simulink model "c00006M_harness"  (R2018a)
settings: Solver=ode3  StartTime=0.0  StopTime=10.0  RelTol=1e-3  EnableMultiTasking=on
undefined symbols (not defined in the file): b, DiscIntNeverNeededParam, J, K, L, PosMinimaW3, R, sigbuilder_block
(part 2 of 42)

== system c00006M_harness/CPSUT ==
  DW1 : Inport  OutMin=0  OutMax=4  OutDataTypeStr=int8
  DW2 : Inport  Port=2  OutMin=0  OutMax=4  OutDataTypeStr=int8
  DW3 : Inport  Port=3  OutMin=0  OutMax=4  OutDataTypeStr=int8
  P1W2 : Inport  Port=4  OutMin=0  OutMax=4  OutDataTypeStr=int8
  P2W3 : Inport  Port=5  OutMin=0  OutMax=4  OutDataTypeStr=int8
  O1 : Inport  Port=6  OutDataTypeStr=boolean
  O2 : Inport  Port=7  OutDataTypeStr=boolean
  O3 : Inport  Port=8  OutDataTypeStr=boolean
  CW3C : Inport  Port=9  OutMin=0  OutMax=4  OutDataTypeStr=int8
  Cyber : Subsystem
  M : Memory
  M1 : Memory
  M2 : Memory
  Physical : Subsystem
  S1 : Subsystem
  S2 : Subsystem
  S3 : Subsystem
  W1Pos : Outport
  W2Pos : Outport  Port=2
  W3Pos : Outport  Port=3
  wires:
  P2W3/1 -> Cyber/8(P2W3)
  S1/1(SensorOut) -> M/1
  CW3C/1 -> Cyber/12(CW3C)
  Physical/1(W1) -> W1Pos/1, S1/1(PhyMeasure)
  S3/1(SensorOut) -> M2/1
  O2/1 -> Cyber/10(OW2)
  Cyber/3(W3) -> Physical/3(InW3)
  O1/1 -> Cyber/9(OW1)
  Cyber/1(W1) -> Physical/1(InW1)
  Cyber/2(W2) -> Physical/2(InW2)
  M2/1 -> Cyber/3(PosW3)
  P1W2/1 -> Cyber/7(P1W2)
  O3/1 -> Cyber/11(OW3)
  DW3/1 -> Cyber/6(DW3)
  M1/1 -> Cyber/2(PosW2)
  Physical/3(W3) -> W3Pos/1, S3/1(PhyMeasure)
  M/1 -> Cyber/1(PosW1)
  DW1/1 -> Cyber/4(DW1)
  Physical/2(W2) -> W2Pos/1, S2/1(PhyMeasure)
  S2/1(SensorOut) -> M1/1
  DW2/1 -> Cyber/5(DW2)

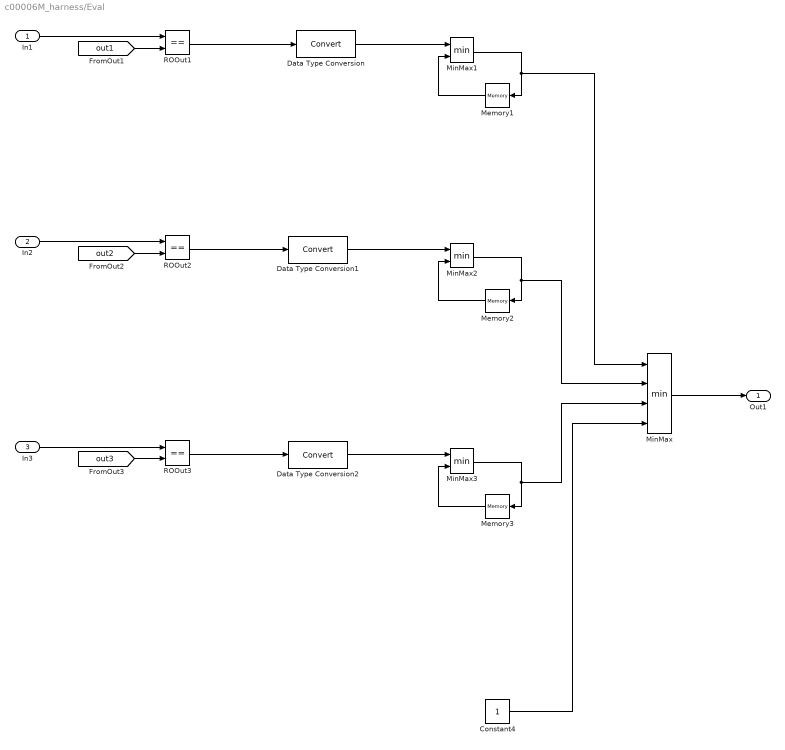
== system c00006M_harness/Eval ==
  In1 : Inport
  In2 : Inport  Port=2
  In3 : Inport  Port=3
  Constant4 : Constant
  Data Type Conversion : DataTypeConversion
  Data Type Conversion1 : DataTypeConversion
  Data Type Conversion2 : DataTypeConversion
  Memory1 : Memory  InitialCondition=1
  Memory2 : Memory  InitialCondition=1
  Memory3 : Memory  InitialCondition=1
  MinMax : MinMax  Inputs=4
  MinMax1 : MinMax  Inputs=2
  MinMax2 : MinMax  Inputs=2
  MinMax3 : MinMax  Inputs=2
  ROOut1 : RelationalOperator  Operator===  OutDataTypeStr=boolean  RndMeth=Simplest
  ROOut2 : RelationalOperator  Operator===  OutDataTypeStr=boolean  RndMeth=Simplest
  ROOut3 : RelationalOperator  Operator===  OutDataTypeStr=boolean  RndMeth=Simplest
  Out1 : Outport
  wires:
  MinMax/1 -> Out1/1
  [out3] -> ROOut3/2
  In3/1 -> ROOut3/1
  [out1] -> ROOut1/2
  In2/1 -> ROOut2/1
  In1/1 -> ROOut1/1
  [out2] -> ROOut2/2
  Memory1/1 -> MinMax1/2
  MinMax3/1 -> MinMax/3, Memory3/1
  ROOut3/1 -> Data Type Conversion2/1
  ROOut2/1 -> Data Type Conversion1/1
  Memory3/1 -> MinMax3/2
  Memory2/1 -> MinMax2/2
  ROOut1/1 -> Data Type Conversion/1
  MinMax2/1 -> MinMax/2, Memory2/1
  MinMax1/1 -> MinMax/1, Memory1/1
  Data Type Conversion/1 -> MinMax1/1
  Data Type Conversion1/1 -> MinMax2/1
  Data Type Conversion2/1 -> MinMax3/1
  Constant4/1 -> MinMax/4

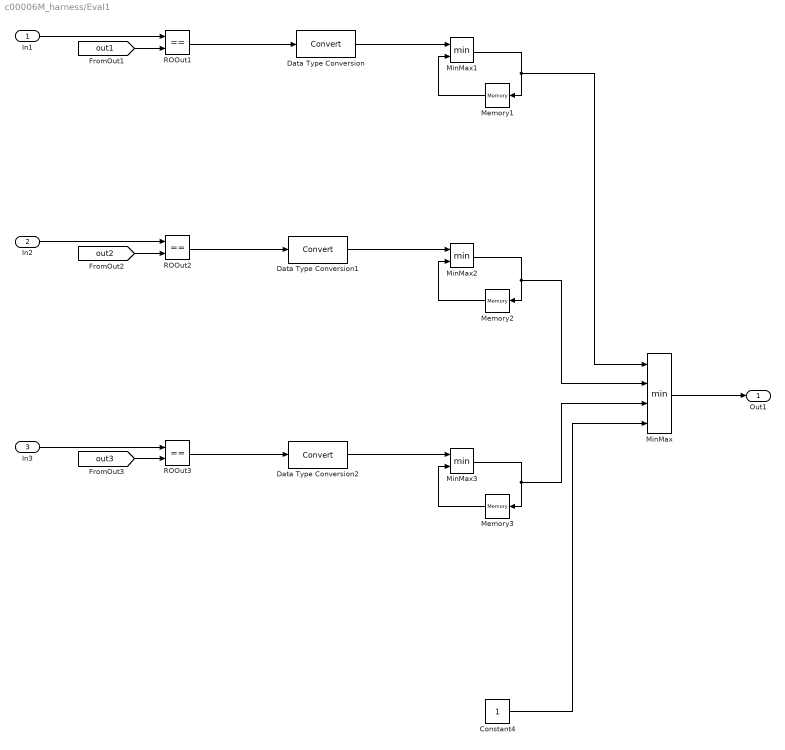
== system c00006M_harness/Eval1 ==
  In1 : Inport
  In2 : Inport  Port=2
  In3 : Inport  Port=3
  Constant4 : Constant
  Data Type Conversion : DataTypeConversion
  Data Type Conversion1 : DataTypeConversion
  Data Type Conversion2 : DataTypeConversion
  Memory1 : Memory  InitialCondition=1
  Memory2 : Memory  InitialCondition=1
  Memory3 : Memory  InitialCondition=1
  MinMax : MinMax  Inputs=4
  MinMax1 : MinMax  Inputs=2
  MinMax2 : MinMax  Inputs=2
  MinMax3 : MinMax  Inputs=2
  ROOut1 : RelationalOperator  Operator===  OutDataTypeStr=boolean  RndMeth=Simplest
  ROOut2 : RelationalOperator  Operator===  OutDataTypeStr=boolean  RndMeth=Simplest
  ROOut3 : RelationalOperator  Operator===  OutDataTypeStr=boolean  RndMeth=Simplest
  Out1 : Outport
  wires:
  Data Type Conversion2/1 -> MinMax3/1
  Data Type Conversion1/1 -> MinMax2/1
  Data Type Conversion/1 -> MinMax1/1
  MinMax1/1 -> Memory1/1, MinMax/1
  MinMax2/1 -> Memory2/1, MinMax/2
  ROOut1/1 -> Data Type Conversion/1
  Memory2/1 -> MinMax2/2
  Memory3/1 -> MinMax3/2
  ROOut2/1 -> Data Type Conversion1/1
  ROOut3/1 -> Data Type Conversion2/1
  MinMax3/1 -> Memory3/1, MinMax/3
  Memory1/1 -> MinMax1/2
  [out2] -> ROOut2/2
  In1/1 -> ROOut1/1
  In2/1 -> ROOut2/1
  [out1] -> ROOut1/2
  In3/1 -> ROOut3/1
  [out3] -> ROOut3/2
  MinMax/1 -> Out1/1
  Constant4/1 -> MinMax/4

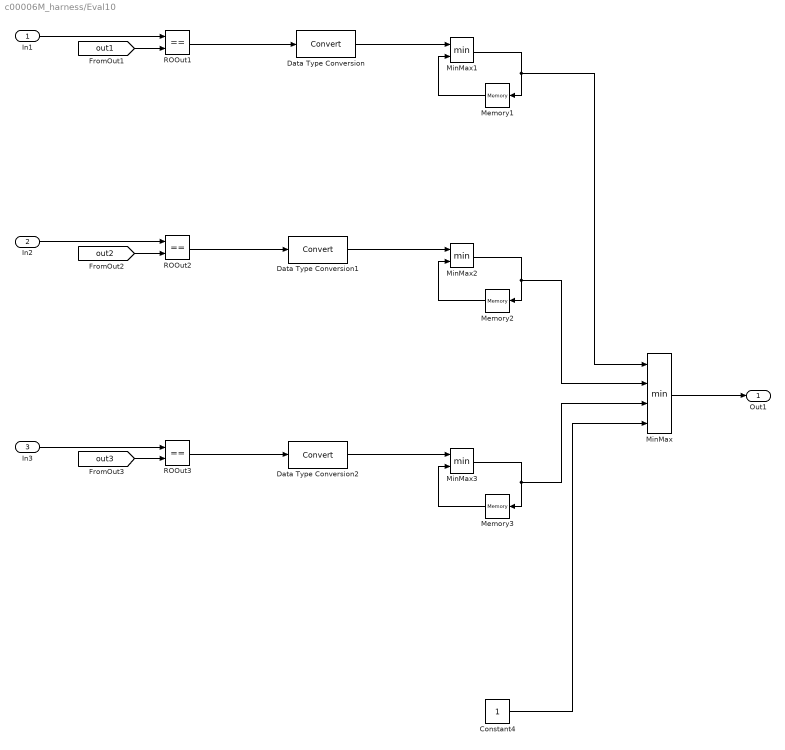
== system c00006M_harness/Eval10 ==
  In1 : Inport
  In2 : Inport  Port=2
  In3 : Inport  Port=3
  Constant4 : Constant
  Data Type Conversion : DataTypeConversion
  Data Type Conversion1 : DataTypeConversion
  Data Type Conversion2 : DataTypeConversion
  Memory1 : Memory  InitialCondition=1
  Memory2 : Memory  InitialCondition=1
  Memory3 : Memory  InitialCondition=1
  MinMax : MinMax  Inputs=4
  MinMax1 : MinMax  Inputs=2
  MinMax2 : MinMax  Inputs=2
  MinMax3 : MinMax  Inputs=2
  ROOut1 : RelationalOperator  Operator===  OutDataTypeStr=boolean  RndMeth=Simplest
  ROOut2 : RelationalOperator  Operator===  OutDataTypeStr=boolean  RndMeth=Simplest
  ROOut3 : RelationalOperator  Operator===  OutDataTypeStr=boolean  RndMeth=Simplest
  Out1 : Outport
  wires:
  Data Type Conversion2/1 -> MinMax3/1
  Data Type Conversion1/1 -> MinMax2/1
  Data Type Conversion/1 -> MinMax1/1
  MinMax1/1 -> Memory1/1, MinMax/1
  MinMax2/1 -> Memory2/1, MinMax/2
  ROOut1/1 -> Data Type Conversion/1
  Memory2/1 -> MinMax2/2
  Memory3/1 -> MinMax3/2
  ROOut2/1 -> Data Type Conversion1/1
  ROOut3/1 -> Data Type Conversion2/1
  MinMax3/1 -> Memory3/1, MinMax/3
  Memory1/1 -> MinMax1/2
  [out2] -> ROOut2/2
  In1/1 -> ROOut1/1
  In2/1 -> ROOut2/1
  [out1] -> ROOut1/2
  In3/1 -> ROOut3/1
  [out3] -> ROOut3/2
  MinMax/1 -> Out1/1
  Constant4/1 -> MinMax/4

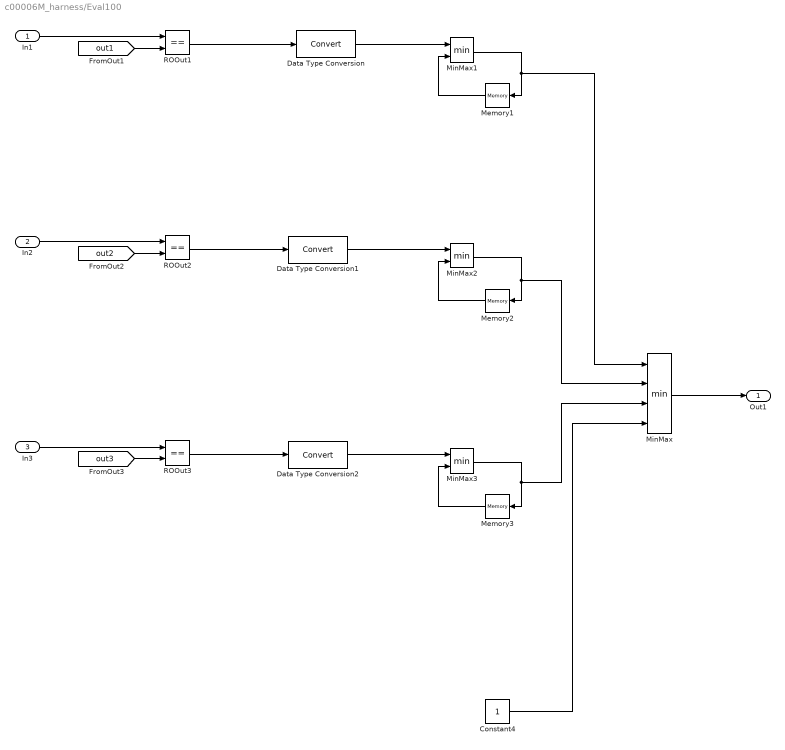
== system c00006M_harness/Eval100 ==
  In1 : Inport
  In2 : Inport  Port=2
  In3 : Inport  Port=3
  Constant4 : Constant
  Data Type Conversion : DataTypeConversion
  Data Type Conversion1 : DataTypeConversion
  Data Type Conversion2 : DataTypeConversion
  Memory1 : Memory  InitialCondition=1
  Memory2 : Memory  InitialCondition=1
  Memory3 : Memory  InitialCondition=1
  MinMax : MinMax  Inputs=4
  MinMax1 : MinMax  Inputs=2
  MinMax2 : MinMax  Inputs=2
  MinMax3 : MinMax  Inputs=2
  ROOut1 : RelationalOperator  Operator===  OutDataTypeStr=boolean  RndMeth=Simplest
  ROOut2 : RelationalOperator  Operator===  OutDataTypeStr=boolean  RndMeth=Simplest
  ROOut3 : RelationalOperator  Operator===  OutDataTypeStr=boolean  RndMeth=Simplest
  Out1 : Outport
  wires:
  Data Type Conversion2/1 -> MinMax3/1
  Data Type Conversion1/1 -> MinMax2/1
  Data Type Conversion/1 -> MinMax1/1
  MinMax1/1 -> Memory1/1, MinMax/1
  MinMax2/1 -> Memory2/1, MinMax/2
  ROOut1/1 -> Data Type Conversion/1
  Memory2/1 -> MinMax2/2
  Memory3/1 -> MinMax3/2
  ROOut2/1 -> Data Type Conversion1/1
  ROOut3/1 -> Data Type Conversion2/1
  MinMax3/1 -> Memory3/1, MinMax/3
  Memory1/1 -> MinMax1/2
  [out2] -> ROOut2/2
  In1/1 -> ROOut1/1
  In2/1 -> ROOut2/1
  [out1] -> ROOut1/2
  In3/1 -> ROOut3/1
  [out3] -> ROOut3/2
  MinMax/1 -> Out1/1
  Constant4/1 -> MinMax/4

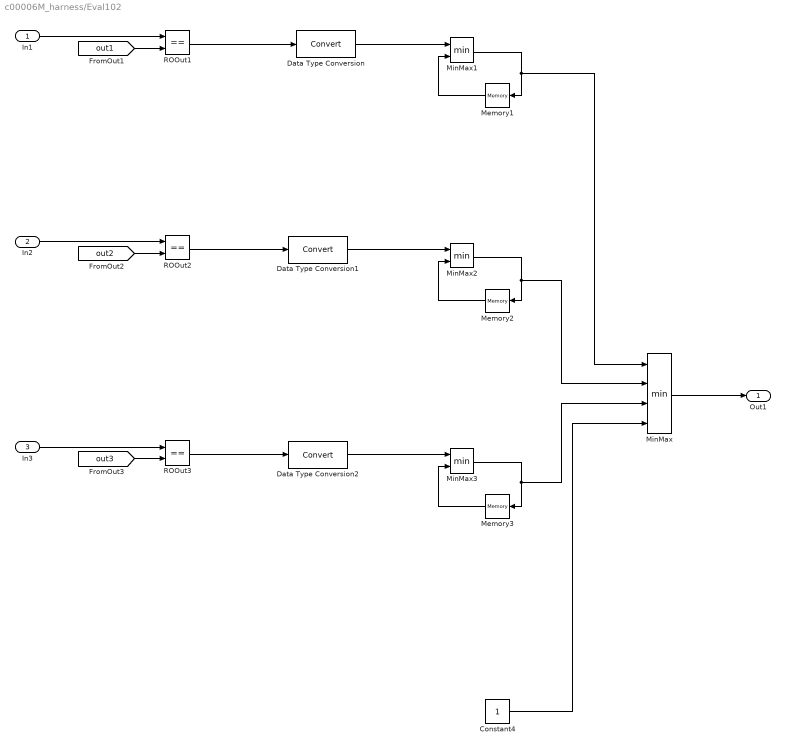
== system c00006M_harness/Eval102 ==
  In1 : Inport
  In2 : Inport  Port=2
  In3 : Inport  Port=3
  Constant4 : Constant
  Data Type Conversion : DataTypeConversion
  Data Type Conversion1 : DataTypeConversion
  Data Type Conversion2 : DataTypeConversion
  Memory1 : Memory  InitialCondition=1
  Memory2 : Memory  InitialCondition=1
  Memory3 : Memory  InitialCondition=1
  MinMax : MinMax  Inputs=4
  MinMax1 : MinMax  Inputs=2
  MinMax2 : MinMax  Inputs=2
  MinMax3 : MinMax  Inputs=2
  ROOut1 : RelationalOperator  Operator===  OutDataTypeStr=boolean  RndMeth=Simplest
  ROOut2 : RelationalOperator  Operator===  OutDataTypeStr=boolean  RndMeth=Simplest
  ROOut3 : RelationalOperator  Operator===  OutDataTypeStr=boolean  RndMeth=Simplest
  Out1 : Outport
  wires:
  Data Type Conversion2/1 -> MinMax3/1
  Data Type Conversion1/1 -> MinMax2/1
  Data Type Conversion/1 -> MinMax1/1
  MinMax1/1 -> Memory1/1, MinMax/1
  MinMax2/1 -> Memory2/1, MinMax/2
  ROOut1/1 -> Data Type Conversion/1
  Memory2/1 -> MinMax2/2
  Memory3/1 -> MinMax3/2
  ROOut2/1 -> Data Type Conversion1/1
  ROOut3/1 -> Data Type Conversion2/1
  MinMax3/1 -> Memory3/1, MinMax/3
  Memory1/1 -> MinMax1/2
  [out2] -> ROOut2/2
  In1/1 -> ROOut1/1
  In2/1 -> ROOut2/1
  [out1] -> ROOut1/2
  In3/1 -> ROOut3/1
  [out3] -> ROOut3/2
  MinMax/1 -> Out1/1
  Constant4/1 -> MinMax/4

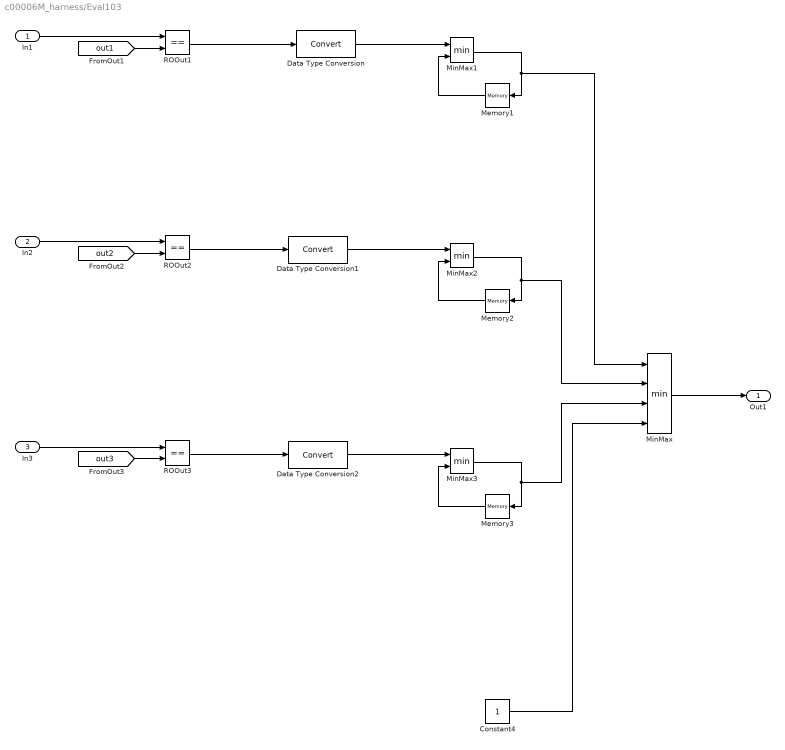
== system c00006M_harness/Eval103 ==
  In1 : Inport
  In2 : Inport  Port=2
  In3 : Inport  Port=3
  Constant4 : Constant
  Data Type Conversion : DataTypeConversion
  Data Type Conversion1 : DataTypeConversion
  Data Type Conversion2 : DataTypeConversion
  Memory1 : Memory  InitialCondition=1
  Memory2 : Memory  InitialCondition=1
  Memory3 : Memory  InitialCondition=1
  MinMax : MinMax  Inputs=4
  MinMax1 : MinMax  Inputs=2
  MinMax2 : MinMax  Inputs=2
  MinMax3 : MinMax  Inputs=2
  ROOut1 : RelationalOperator  Operator===  OutDataTypeStr=boolean  RndMeth=Simplest
  ROOut2 : RelationalOperator  Operator===  OutDataTypeStr=boolean  RndMeth=Simplest
  ROOut3 : RelationalOperator  Operator===  OutDataTypeStr=boolean  RndMeth=Simplest
  Out1 : Outport
  wires:
  Data Type Conversion2/1 -> MinMax3/1
  Data Type Conversion1/1 -> MinMax2/1
  Data Type Conversion/1 -> MinMax1/1
  MinMax1/1 -> Memory1/1, MinMax/1
  MinMax2/1 -> Memory2/1, MinMax/2
  ROOut1/1 -> Data Type Conversion/1
  Memory2/1 -> MinMax2/2
  Memory3/1 -> MinMax3/2
  ROOut2/1 -> Data Type Conversion1/1
  ROOut3/1 -> Data Type Conversion2/1
  MinMax3/1 -> Memory3/1, MinMax/3
  Memory1/1 -> MinMax1/2
  [out2] -> ROOut2/2
  In1/1 -> ROOut1/1
  In2/1 -> ROOut2/1
  [out1] -> ROOut1/2
  In3/1 -> ROOut3/1
  [out3] -> ROOut3/2
  MinMax/1 -> Out1/1
  Constant4/1 -> MinMax/4

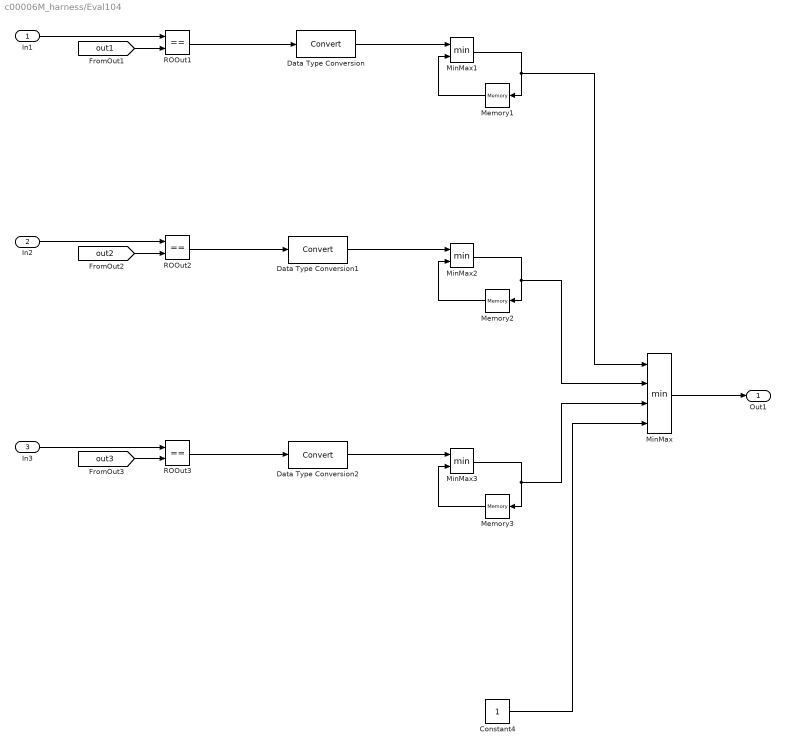
== system c00006M_harness/Eval104 ==
  In1 : Inport
  In2 : Inport  Port=2
  In3 : Inport  Port=3
  Constant4 : Constant
  Data Type Conversion : DataTypeConversion
  Data Type Conversion1 : DataTypeConversion
  Data Type Conversion2 : DataTypeConversion
  Memory1 : Memory  InitialCondition=1
  Memory2 : Memory  InitialCondition=1
  Memory3 : Memory  InitialCondition=1
  MinMax : MinMax  Inputs=4
  MinMax1 : MinMax  Inputs=2
  MinMax2 : MinMax  Inputs=2
  MinMax3 : MinMax  Inputs=2
  ROOut1 : RelationalOperator  Operator===  OutDataTypeStr=boolean  RndMeth=Simplest
  ROOut2 : RelationalOperator  Operator===  OutDataTypeStr=boolean  RndMeth=Simplest
  ROOut3 : RelationalOperator  Operator===  OutDataTypeStr=boolean  RndMeth=Simplest
  Out1 : Outport
  wires:
  Data Type Conversion2/1 -> MinMax3/1
  Data Type Conversion1/1 -> MinMax2/1
  Data Type Conversion/1 -> MinMax1/1
  MinMax1/1 -> Memory1/1, MinMax/1
  MinMax2/1 -> Memory2/1, MinMax/2
  ROOut1/1 -> Data Type Conversion/1
  Memory2/1 -> MinMax2/2
  Memory3/1 -> MinMax3/2
  ROOut2/1 -> Data Type Conversion1/1
  ROOut3/1 -> Data Type Conversion2/1
  MinMax3/1 -> Memory3/1, MinMax/3
  Memory1/1 -> MinMax1/2
  [out2] -> ROOut2/2
  In1/1 -> ROOut1/1
  In2/1 -> ROOut2/1
  [out1] -> ROOut1/2
  In3/1 -> ROOut3/1
  [out3] -> ROOut3/2
  MinMax/1 -> Out1/1
  Constant4/1 -> MinMax/4

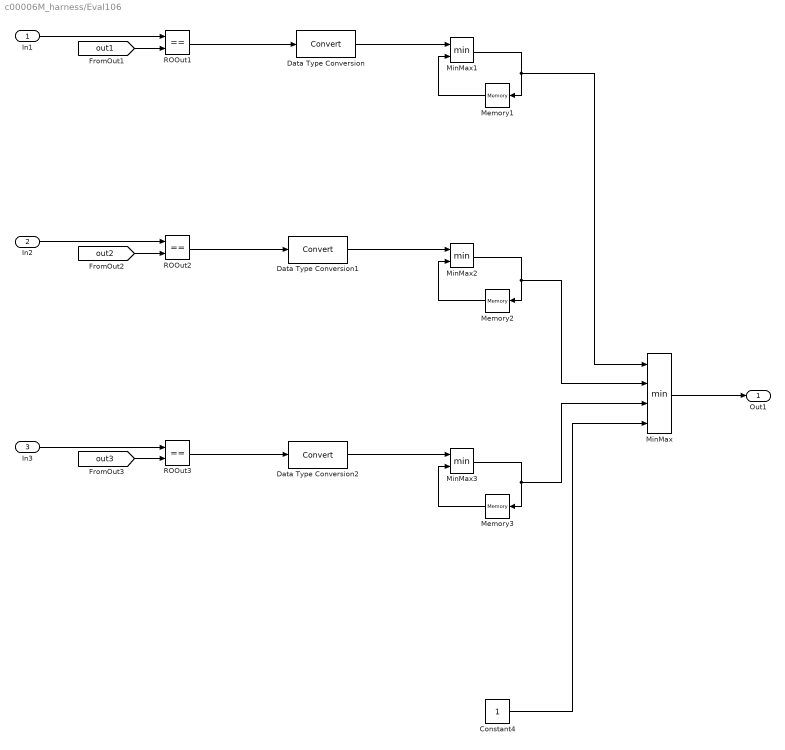
== system c00006M_harness/Eval106 ==
  In1 : Inport
  In2 : Inport  Port=2
  In3 : Inport  Port=3
  Constant4 : Constant
  Data Type Conversion : DataTypeConversion
  Data Type Conversion1 : DataTypeConversion
  Data Type Conversion2 : DataTypeConversion
  Memory1 : Memory  InitialCondition=1
  Memory2 : Memory  InitialCondition=1
  Memory3 : Memory  InitialCondition=1
  MinMax : MinMax  Inputs=4
  MinMax1 : MinMax  Inputs=2
  MinMax2 : MinMax  Inputs=2
  MinMax3 : MinMax  Inputs=2
  ROOut1 : RelationalOperator  Operator===  OutDataTypeStr=boolean  RndMeth=Simplest
  ROOut2 : RelationalOperator  Operator===  OutDataTypeStr=boolean  RndMeth=Simplest
  ROOut3 : RelationalOperator  Operator===  OutDataTypeStr=boolean  RndMeth=Simplest
  Out1 : Outport
  wires:
  Data Type Conversion2/1 -> MinMax3/1
  Data Type Conversion1/1 -> MinMax2/1
  Data Type Conversion/1 -> MinMax1/1
  MinMax1/1 -> Memory1/1, MinMax/1
  MinMax2/1 -> Memory2/1, MinMax/2
  ROOut1/1 -> Data Type Conversion/1
  Memory2/1 -> MinMax2/2
  Memory3/1 -> MinMax3/2
  ROOut2/1 -> Data Type Conversion1/1
  ROOut3/1 -> Data Type Conversion2/1
  MinMax3/1 -> Memory3/1, MinMax/3
  Memory1/1 -> MinMax1/2
  [out2] -> ROOut2/2
  In1/1 -> ROOut1/1
  In2/1 -> ROOut2/1
  [out1] -> ROOut1/2
  In3/1 -> ROOut3/1
  [out3] -> ROOut3/2
  MinMax/1 -> Out1/1
  Constant4/1 -> MinMax/4

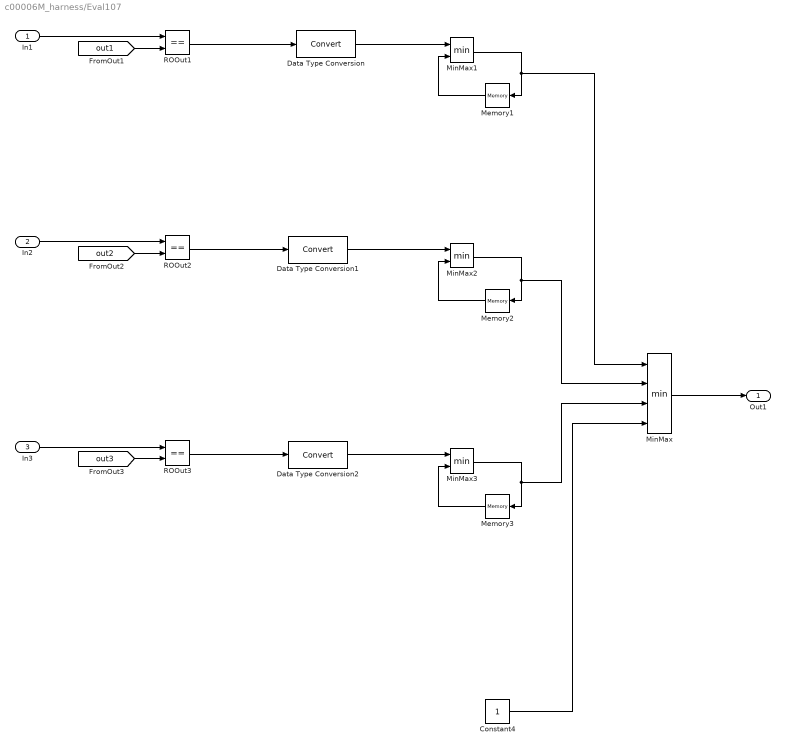
== system c00006M_harness/Eval107 ==
  In1 : Inport
  In2 : Inport  Port=2
  In3 : Inport  Port=3
  Constant4 : Constant
  Data Type Conversion : DataTypeConversion
  Data Type Conversion1 : DataTypeConversion
  Data Type Conversion2 : DataTypeConversion
  Memory1 : Memory  InitialCondition=1
  Memory2 : Memory  InitialCondition=1
  Memory3 : Memory  InitialCondition=1
  MinMax : MinMax  Inputs=4
  MinMax1 : MinMax  Inputs=2
  MinMax2 : MinMax  Inputs=2
  MinMax3 : MinMax  Inputs=2
  ROOut1 : RelationalOperator  Operator===  OutDataTypeStr=boolean  RndMeth=Simplest
  ROOut2 : RelationalOperator  Operator===  OutDataTypeStr=boolean  RndMeth=Simplest
  ROOut3 : RelationalOperator  Operator===  OutDataTypeStr=boolean  RndMeth=Simplest
  Out1 : Outport
  wires:
  Data Type Conversion2/1 -> MinMax3/1
  Data Type Conversion1/1 -> MinMax2/1
  Data Type Conversion/1 -> MinMax1/1
  MinMax1/1 -> Memory1/1, MinMax/1
  MinMax2/1 -> Memory2/1, MinMax/2
  ROOut1/1 -> Data Type Conversion/1
  Memory2/1 -> MinMax2/2
  Memory3/1 -> MinMax3/2
  ROOut2/1 -> Data Type Conversion1/1
  ROOut3/1 -> Data Type Conversion2/1
  MinMax3/1 -> Memory3/1, MinMax/3
  Memory1/1 -> MinMax1/2
  [out2] -> ROOut2/2
  In1/1 -> ROOut1/1
  In2/1 -> ROOut2/1
  [out1] -> ROOut1/2
  In3/1 -> ROOut3/1
  [out3] -> ROOut3/2
  MinMax/1 -> Out1/1
  Constant4/1 -> MinMax/4

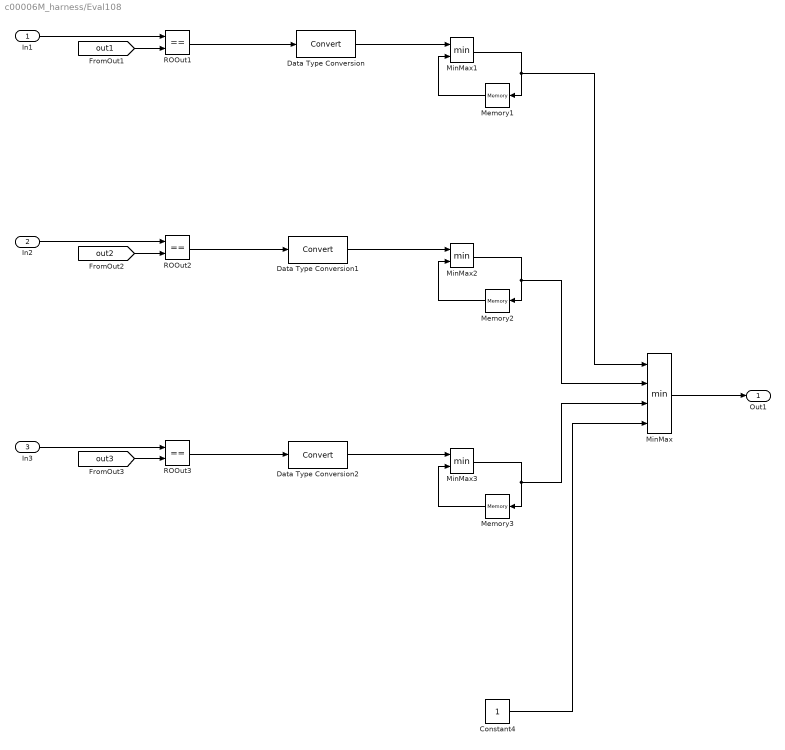
== system c00006M_harness/Eval108 ==
  In1 : Inport
  In2 : Inport  Port=2
  In3 : Inport  Port=3
  Constant4 : Constant
  Data Type Conversion : DataTypeConversion
  Data Type Conversion1 : DataTypeConversion
  Data Type Conversion2 : DataTypeConversion
  Memory1 : Memory  InitialCondition=1
  Memory2 : Memory  InitialCondition=1
  Memory3 : Memory  InitialCondition=1
  MinMax : MinMax  Inputs=4
  MinMax1 : MinMax  Inputs=2
  MinMax2 : MinMax  Inputs=2
  MinMax3 : MinMax  Inputs=2
  ROOut1 : RelationalOperator  Operator===  OutDataTypeStr=boolean  RndMeth=Simplest
  ROOut2 : RelationalOperator  Operator===  OutDataTypeStr=boolean  RndMeth=Simplest
  ROOut3 : RelationalOperator  Operator===  OutDataTypeStr=boolean  RndMeth=Simplest
  Out1 : Outport
  wires:
  Data Type Conversion2/1 -> MinMax3/1
  Data Type Conversion1/1 -> MinMax2/1
  Data Type Conversion/1 -> MinMax1/1
  MinMax1/1 -> Memory1/1, MinMax/1
  MinMax2/1 -> Memory2/1, MinMax/2
  ROOut1/1 -> Data Type Conversion/1
  Memory2/1 -> MinMax2/2
  Memory3/1 -> MinMax3/2
  ROOut2/1 -> Data Type Conversion1/1
  ROOut3/1 -> Data Type Conversion2/1
  MinMax3/1 -> Memory3/1, MinMax/3
  Memory1/1 -> MinMax1/2
  [out2] -> ROOut2/2
  In1/1 -> ROOut1/1
  In2/1 -> ROOut2/1
  [out1] -> ROOut1/2
  In3/1 -> ROOut3/1
  [out3] -> ROOut3/2
  MinMax/1 -> Out1/1
  Constant4/1 -> MinMax/4

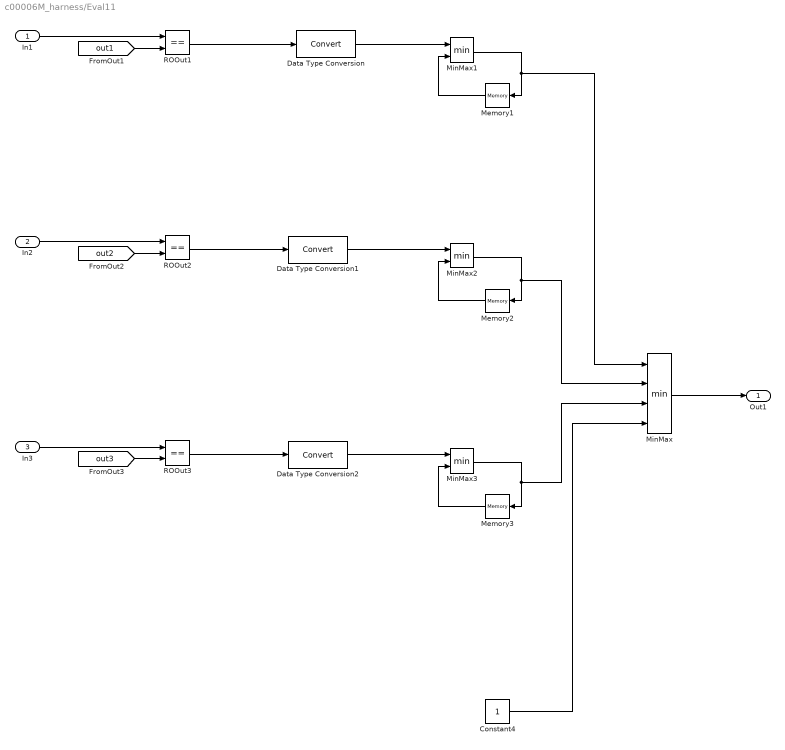
== system c00006M_harness/Eval11 ==
  In1 : Inport
  In2 : Inport  Port=2
  In3 : Inport  Port=3
  Constant4 : Constant
  Data Type Conversion : DataTypeConversion
  Data Type Conversion1 : DataTypeConversion
  Data Type Conversion2 : DataTypeConversion
  Memory1 : Memory  InitialCondition=1
  Memory2 : Memory  InitialCondition=1
  Memory3 : Memory  InitialCondition=1
  MinMax : MinMax  Inputs=4
  MinMax1 : MinMax  Inputs=2
  MinMax2 : MinMax  Inputs=2
  MinMax3 : MinMax  Inputs=2
  ROOut1 : RelationalOperator  Operator===  OutDataTypeStr=boolean  RndMeth=Simplest
  ROOut2 : RelationalOperator  Operator===  OutDataTypeStr=boolean  RndMeth=Simplest
  ROOut3 : RelationalOperator  Operator===  OutDataTypeStr=boolean  RndMeth=Simplest
  Out1 : Outport
  wires:
  Data Type Conversion2/1 -> MinMax3/1
  Data Type Conversion1/1 -> MinMax2/1
  Data Type Conversion/1 -> MinMax1/1
  MinMax1/1 -> Memory1/1, MinMax/1
  MinMax2/1 -> Memory2/1, MinMax/2
  ROOut1/1 -> Data Type Conversion/1
  Memory2/1 -> MinMax2/2
  Memory3/1 -> MinMax3/2
  ROOut2/1 -> Data Type Conversion1/1
  ROOut3/1 -> Data Type Conversion2/1
  MinMax3/1 -> Memory3/1, MinMax/3
  Memory1/1 -> MinMax1/2
  [out2] -> ROOut2/2
  In1/1 -> ROOut1/1
  In2/1 -> ROOut2/1
  [out1] -> ROOut1/2
  In3/1 -> ROOut3/1
  [out3] -> ROOut3/2
  MinMax/1 -> Out1/1
  Constant4/1 -> MinMax/4

== system c00006M_harness/Eval110 ==
  In1 : Inport
  In2 : Inport  Port=2
  In3 : Inport  Port=3
  Constant4 : Constant
  Data Type Conversion : DataTypeConversion
  Data Type Conversion1 : DataTypeConversion
  Data Type Conversion2 : DataTypeConversion
  Memory1 : Memory  InitialCondition=1
  Memory2 : Memory  InitialCondition=1
  Memory3 : Memory  InitialCondition=1
  MinMax : MinMax  Inputs=4
  MinMax1 : MinMax  Inputs=2
  MinMax2 : MinMax  Inputs=2
  MinMax3 : MinMax  Inputs=2
  ROOut1 : RelationalOperator  Operator===  OutDataTypeStr=boolean  RndMeth=Simplest
  ROOut2 : RelationalOperator  Operator===  OutDataTypeStr=boolean  RndMeth=Simplest
  ROOut3 : RelationalOperator  Operator===  OutDataTypeStr=boolean  RndMeth=Simplest
  Out1 : Outport
  wires:
  Data Type Conversion2/1 -> MinMax3/1
  Data Type Conversion1/1 -> MinMax2/1
  Data Type Conversion/1 -> MinMax1/1
  MinMax1/1 -> Memory1/1, MinMax/1
  MinMax2/1 -> Memory2/1, MinMax/2
  ROOut1/1 -> Data Type Conversion/1
  Memory2/1 -> MinMax2/2
  Memory3/1 -> MinMax3/2
  ROOut2/1 -> Data Type Conversion1/1
  ROOut3/1 -> Data Type Conversion2/1
  MinMax3/1 -> Memory3/1, MinMax/3
  Memory1/1 -> MinMax1/2
  [out2] -> ROOut2/2
  In1/1 -> ROOut1/1
  In2/1 -> ROOut2/1
  [out1] -> ROOut1/2
  In3/1 -> ROOut3/1
  [out3] -> ROOut3/2
  MinMax/1 -> Out1/1
  Constant4/1 -> MinMax/4

== system c00006M_harness/Eval111 ==
  In1 : Inport
  In2 : Inport  Port=2
  In3 : Inport  Port=3
  Constant4 : Constant
  Data Type Conversion : DataTypeConversion
  Data Type Conversion1 : DataTypeConversion
  Data Type Conversion2 : DataTypeConversion
  Memory1 : Memory  InitialCondition=1
  Memory2 : Memory  InitialCondition=1
  Memory3 : Memory  InitialCondition=1
  MinMax : MinMax  Inputs=4
  MinMax1 : MinMax  Inputs=2
  MinMax2 : MinMax  Inputs=2
  MinMax3 : MinMax  Inputs=2
  ROOut1 : RelationalOperator  Operator===  OutDataTypeStr=boolean  RndMeth=Simplest
  ROOut2 : RelationalOperator  Operator===  OutDataTypeStr=boolean  RndMeth=Simplest
  ROOut3 : RelationalOperator  Operator===  OutDataTypeStr=boolean  RndMeth=Simplest
  Out1 : Outport
  wires:
  Data Type Conversion2/1 -> MinMax3/1
  Data Type Conversion1/1 -> MinMax2/1
  Data Type Conversion/1 -> MinMax1/1
  MinMax1/1 -> Memory1/1, MinMax/1
  MinMax2/1 -> Memory2/1, MinMax/2
  ROOut1/1 -> Data Type Conversion/1
  Memory2/1 -> MinMax2/2
  Memory3/1 -> MinMax3/2
  ROOut2/1 -> Data Type Conversion1/1
  ROOut3/1 -> Data Type Conversion2/1
  MinMax3/1 -> Memory3/1, MinMax/3
  Memory1/1 -> MinMax1/2
  [out2] -> ROOut2/2
  In1/1 -> ROOut1/1
  In2/1 -> ROOut2/1
  [out1] -> ROOut1/2
  In3/1 -> ROOut3/1
  [out3] -> ROOut3/2
  MinMax/1 -> Out1/1
  Constant4/1 -> MinMax/4

== system c00006M_harness/Eval112 ==
  In1 : Inport
  In2 : Inport  Port=2
  In3 : Inport  Port=3
  Constant4 : Constant
  Data Type Conversion : DataTypeConversion
  Data Type Conversion1 : DataTypeConversion
  Data Type Conversion2 : DataTypeConversion
  Memory1 : Memory  InitialCondition=1
  Memory2 : Memory  InitialCondition=1
  Memory3 : Memory  InitialCondition=1
  MinMax : MinMax  Inputs=4
  MinMax1 : MinMax  Inputs=2
  MinMax2 : MinMax  Inputs=2
  MinMax3 : MinMax  Inputs=2
  ROOut1 : RelationalOperator  Operator===  OutDataTypeStr=boolean  RndMeth=Simplest
  ROOut2 : RelationalOperator  Operator===  OutDataTypeStr=boolean  RndMeth=Simplest
  ROOut3 : RelationalOperator  Operator===  OutDataTypeStr=boolean  RndMeth=Simplest
  Out1 : Outport
  wires:
  Data Type Conversion2/1 -> MinMax3/1
  Data Type Conversion1/1 -> MinMax2/1
  Data Type Conversion/1 -> MinMax1/1
  MinMax1/1 -> Memory1/1, MinMax/1
  MinMax2/1 -> Memory2/1, MinMax/2
  ROOut1/1 -> Data Type Conversion/1
  Memory2/1 -> MinMax2/2
  Memory3/1 -> MinMax3/2
  ROOut2/1 -> Data Type Conversion1/1
  ROOut3/1 -> Data Type Conversion2/1
  MinMax3/1 -> Memory3/1, MinMax/3
  Memory1/1 -> MinMax1/2
  [out2] -> ROOut2/2
  In1/1 -> ROOut1/1
  In2/1 -> ROOut2/1
  [out1] -> ROOut1/2
  In3/1 -> ROOut3/1
  [out3] -> ROOut3/2
  MinMax/1 -> Out1/1
  Constant4/1 -> MinMax/4

== system c00006M_harness/Eval114 ==
  In1 : Inport
  In2 : Inport  Port=2
  In3 : Inport  Port=3
  Constant4 : Constant
  Data Type Conversion : DataTypeConversion
  Data Type Conversion1 : DataTypeConversion
  Data Type Conversion2 : DataTypeConversion
  Memory1 : Memory  InitialCondition=1
  Memory2 : Memory  InitialCondition=1
  Memory3 : Memory  InitialCondition=1
  MinMax : MinMax  Inputs=4
  MinMax1 : MinMax  Inputs=2
  MinMax2 : MinMax  Inputs=2
  MinMax3 : MinMax  Inputs=2
  ROOut1 : RelationalOperator  Operator===  OutDataTypeStr=boolean  RndMeth=Simplest
  ROOut2 : RelationalOperator  Operator===  OutDataTypeStr=boolean  RndMeth=Simplest
  ROOut3 : RelationalOperator  Operator===  OutDataTypeStr=boolean  RndMeth=Simplest
  Out1 : Outport
  wires:
  Data Type Conversion2/1 -> MinMax3/1
  Data Type Conversion1/1 -> MinMax2/1
  Data Type Conversion/1 -> MinMax1/1
  MinMax1/1 -> Memory1/1, MinMax/1
  MinMax2/1 -> Memory2/1, MinMax/2
  ROOut1/1 -> Data Type Conversion/1
  Memory2/1 -> MinMax2/2
  Memory3/1 -> MinMax3/2
  ROOut2/1 -> Data Type Conversion1/1
  ROOut3/1 -> Data Type Conversion2/1
  MinMax3/1 -> Memory3/1, MinMax/3
  Memory1/1 -> MinMax1/2
  [out2] -> ROOut2/2
  In1/1 -> ROOut1/1
  In2/1 -> ROOut2/1
  [out1] -> ROOut1/2
  In3/1 -> ROOut3/1
  [out3] -> ROOut3/2
  MinMax/1 -> Out1/1
  Constant4/1 -> MinMax/4

== system c00006M_harness/Eval115 ==
  In1 : Inport
  In2 : Inport  Port=2
  In3 : Inport  Port=3
  Constant4 : Constant
  Data Type Conversion : DataTypeConversion
  Data Type Conversion1 : DataTypeConversion
  Data Type Conversion2 : DataTypeConversion
  Memory1 : Memory  InitialCondition=1
  Memory2 : Memory  InitialCondition=1
  Memory3 : Memory  InitialCondition=1
  MinMax : MinMax  Inputs=4
  MinMax1 : MinMax  Inputs=2
  MinMax2 : MinMax  Inputs=2
  MinMax3 : MinMax  Inputs=2
  ROOut1 : RelationalOperator  Operator===  OutDataTypeStr=boolean  RndMeth=Simplest
  ROOut2 : RelationalOperator  Operator===  OutDataTypeStr=boolean  RndMeth=Simplest
  ROOut3 : RelationalOperator  Operator===  OutDataTypeStr=boolean  RndMeth=Simplest
  Out1 : Outport
  wires:
  Data Type Conversion2/1 -> MinMax3/1
  Data Type Conversion1/1 -> MinMax2/1
  Data Type Conversion/1 -> MinMax1/1
  MinMax1/1 -> Memory1/1, MinMax/1
  MinMax2/1 -> Memory2/1, MinMax/2
  ROOut1/1 -> Data Type Conversion/1
  Memory2/1 -> MinMax2/2
  Memory3/1 -> MinMax3/2
  ROOut2/1 -> Data Type Conversion1/1
  ROOut3/1 -> Data Type Conversion2/1
  MinMax3/1 -> Memory3/1, MinMax/3
  Memory1/1 -> MinMax1/2
  [out2] -> ROOut2/2
  In1/1 -> ROOut1/1
  In2/1 -> ROOut2/1
  [out1] -> ROOut1/2
  In3/1 -> ROOut3/1
  [out3] -> ROOut3/2
  MinMax/1 -> Out1/1
  Constant4/1 -> MinMax/4

== system c00006M_harness/Eval116 ==
  In1 : Inport
  In2 : Inport  Port=2
  In3 : Inport  Port=3
  Constant4 : Constant
  Data Type Conversion : DataTypeConversion
  Data Type Conversion1 : DataTypeConversion
  Data Type Conversion2 : DataTypeConversion
  Memory1 : Memory  InitialCondition=1
  Memory2 : Memory  InitialCondition=1
  Memory3 : Memory  InitialCondition=1
  MinMax : MinMax  Inputs=4
  MinMax1 : MinMax  Inputs=2
  MinMax2 : MinMax  Inputs=2
  MinMax3 : MinMax  Inputs=2
  ROOut1 : RelationalOperator  Operator===  OutDataTypeStr=boolean  RndMeth=Simplest
  ROOut2 : RelationalOperator  Operator===  OutDataTypeStr=boolean  RndMeth=Simplest
  ROOut3 : RelationalOperator  Operator===  OutDataTypeStr=boolean  RndMeth=Simplest
  Out1 : Outport
  wires:
  Data Type Conversion2/1 -> MinMax3/1
  Data Type Conversion1/1 -> MinMax2/1
  Data Type Conversion/1 -> MinMax1/1
  MinMax1/1 -> Memory1/1, MinMax/1
  MinMax2/1 -> Memory2/1, MinMax/2
  ROOut1/1 -> Data Type Conversion/1
  Memory2/1 -> MinMax2/2
  Memory3/1 -> MinMax3/2
  ROOut2/1 -> Data Type Conversion1/1
  ROOut3/1 -> Data Type Conversion2/1
  MinMax3/1 -> Memory3/1, MinMax/3
  Memory1/1 -> MinMax1/2
  [out2] -> ROOut2/2
  In1/1 -> ROOut1/1
  In2/1 -> ROOut2/1
  [out1] -> ROOut1/2
  In3/1 -> ROOut3/1
  [out3] -> ROOut3/2
  MinMax/1 -> Out1/1
  Constant4/1 -> MinMax/4

== system c00006M_harness/Eval118 ==
  In1 : Inport
  In2 : Inport  Port=2
  In3 : Inport  Port=3
  Constant4 : Constant
  Data Type Conversion : DataTypeConversion
  Data Type Conversion1 : DataTypeConversion
  Data Type Conversion2 : DataTypeConversion
  Memory1 : Memory  InitialCondition=1
  Memory2 : Memory  InitialCondition=1
  Memory3 : Memory  InitialCondition=1
  MinMax : MinMax  Inputs=4
  MinMax1 : MinMax  Inputs=2
  MinMax2 : MinMax  Inputs=2
  MinMax3 : MinMax  Inputs=2
  ROOut1 : RelationalOperator  Operator===  OutDataTypeStr=boolean  RndMeth=Simplest
  ROOut2 : RelationalOperator  Operator===  OutDataTypeStr=boolean  RndMeth=Simplest
  ROOut3 : RelationalOperator  Operator===  OutDataTypeStr=boolean  RndMeth=Simplest
  Out1 : Outport
  wires:
  Data Type Conversion2/1 -> MinMax3/1
  Data Type Conversion1/1 -> MinMax2/1
  Data Type Conversion/1 -> MinMax1/1
  MinMax1/1 -> Memory1/1, MinMax/1
  MinMax2/1 -> Memory2/1, MinMax/2
  ROOut1/1 -> Data Type Conversion/1
  Memory2/1 -> MinMax2/2
  Memory3/1 -> MinMax3/2
  ROOut2/1 -> Data Type Conversion1/1
  ROOut3/1 -> Data Type Conversion2/1
  MinMax3/1 -> Memory3/1, MinMax/3
  Memory1/1 -> MinMax1/2
  [out2] -> ROOut2/2
  In1/1 -> ROOut1/1
  In2/1 -> ROOut2/1
  [out1] -> ROOut1/2
  In3/1 -> ROOut3/1
  [out3] -> ROOut3/2
  MinMax/1 -> Out1/1
  Constant4/1 -> MinMax/4

== system c00006M_harness/Eval119 ==
  In1 : Inport
  In2 : Inport  Port=2
  In3 : Inport  Port=3
  Constant4 : Constant
  Data Type Conversion : DataTypeConversion
  Data Type Conversion1 : DataTypeConversion
  Data Type Conversion2 : DataTypeConversion
  Memory1 : Memory  InitialCondition=1
  Memory2 : Memory  InitialCondition=1
  Memory3 : Memory  InitialCondition=1
  MinMax : MinMax  Inputs=4
  MinMax1 : MinMax  Inputs=2
  MinMax2 : MinMax  Inputs=2
  MinMax3 : MinMax  Inputs=2
  ROOut1 : RelationalOperator  Operator===  OutDataTypeStr=boolean  RndMeth=Simplest
  ROOut2 : RelationalOperator  Operator===  OutDataTypeStr=boolean  RndMeth=Simplest
  ROOut3 : RelationalOperator  Operator===  OutDataTypeStr=boolean  RndMeth=Simplest
  Out1 : Outport
  wires:
  Data Type Conversion2/1 -> MinMax3/1
  Data Type Conversion1/1 -> MinMax2/1
  Data Type Conversion/1 -> MinMax1/1
  MinMax1/1 -> Memory1/1, MinMax/1
  MinMax2/1 -> Memory2/1, MinMax/2
  ROOut1/1 -> Data Type Conversion/1
  Memory2/1 -> MinMax2/2
  Memory3/1 -> MinMax3/2
  ROOut2/1 -> Data Type Conversion1/1
  ROOut3/1 -> Data Type Conversion2/1
  MinMax3/1 -> Memory3/1, MinMax/3
  Memory1/1 -> MinMax1/2
  [out2] -> ROOut2/2
  In1/1 -> ROOut1/1
  In2/1 -> ROOut2/1
  [out1] -> ROOut1/2
  In3/1 -> ROOut3/1
  [out3] -> ROOut3/2
  MinMax/1 -> Out1/1
  Constant4/1 -> MinMax/4

== system c00006M_harness/Eval12 ==
  In1 : Inport
  In2 : Inport  Port=2
  In3 : Inport  Port=3
  Constant4 : Constant
  Data Type Conversion : DataTypeConversion
  Data Type Conversion1 : DataTypeConversion
  Data Type Conversion2 : DataTypeConversion
  Memory1 : Memory  InitialCondition=1
  Memory2 : Memory  InitialCondition=1
  Memory3 : Memory  InitialCondition=1
  MinMax : MinMax  Inputs=4
  MinMax1 : MinMax  Inputs=2
  MinMax2 : MinMax  Inputs=2
  MinMax3 : MinMax  Inputs=2
  ROOut1 : RelationalOperator  Operator===  OutDataTypeStr=boolean  RndMeth=Simplest
  ROOut2 : RelationalOperator  Operator===  OutDataTypeStr=boolean  RndMeth=Simplest
  ROOut3 : RelationalOperator  Operator===  OutDataTypeStr=boolean  RndMeth=Simplest
  Out1 : Outport
  wires:
  Data Type Conversion2/1 -> MinMax3/1
  Data Type Conversion1/1 -> MinMax2/1
  Data Type Conversion/1 -> MinMax1/1
  MinMax1/1 -> Memory1/1, MinMax/1
  MinMax2/1 -> Memory2/1, MinMax/2
  ROOut1/1 -> Data Type Conversion/1
  Memory2/1 -> MinMax2/2
  Memory3/1 -> MinMax3/2
  ROOut2/1 -> Data Type Conversion1/1
  ROOut3/1 -> Data Type Conversion2/1
  MinMax3/1 -> Memory3/1, MinMax/3
  Memory1/1 -> MinMax1/2
  [out2] -> ROOut2/2
  In1/1 -> ROOut1/1
  In2/1 -> ROOut2/1
  [out1] -> ROOut1/2
  In3/1 -> ROOut3/1
  [out3] -> ROOut3/2
  MinMax/1 -> Out1/1
  Constant4/1 -> MinMax/4

== system c00006M_harness/Eval120 ==
  In1 : Inport
  In2 : Inport  Port=2
  In3 : Inport  Port=3
  Constant4 : Constant
  Data Type Conversion : DataTypeConversion
  Data Type Conversion1 : DataTypeConversion
  Data Type Conversion2 : DataTypeConversion
  Memory1 : Memory  InitialCondition=1
  Memory2 : Memory  InitialCondition=1
  Memory3 : Memory  InitialCondition=1
  MinMax : MinMax  Inputs=4
  MinMax1 : MinMax  Inputs=2
  MinMax2 : MinMax  Inputs=2
  MinMax3 : MinMax  Inputs=2
  ROOut1 : RelationalOperator  Operator===  OutDataTypeStr=boolean  RndMeth=Simplest
  ROOut2 : RelationalOperator  Operator===  OutDataTypeStr=boolean  RndMeth=Simplest
  ROOut3 : RelationalOperator  Operator===  OutDataTypeStr=boolean  RndMeth=Simplest
  Out1 : Outport
  wires:
  Data Type Conversion2/1 -> MinMax3/1
  Data Type Conversion1/1 -> MinMax2/1
  Data Type Conversion/1 -> MinMax1/1
  MinMax1/1 -> Memory1/1, MinMax/1
  MinMax2/1 -> Memory2/1, MinMax/2
  ROOut1/1 -> Data Type Conversion/1
  Memory2/1 -> MinMax2/2
  Memory3/1 -> MinMax3/2
  ROOut2/1 -> Data Type Conversion1/1
  ROOut3/1 -> Data Type Conversion2/1
  MinMax3/1 -> Memory3/1, MinMax/3
  Memory1/1 -> MinMax1/2
  [out2] -> ROOut2/2
  In1/1 -> ROOut1/1
  In2/1 -> ROOut2/1
  [out1] -> ROOut1/2
  In3/1 -> ROOut3/1
  [out3] -> ROOut3/2
  MinMax/1 -> Out1/1
  Constant4/1 -> MinMax/4

== system c00006M_harness/Eval122 ==
  In1 : Inport
  In2 : Inport  Port=2
  In3 : Inport  Port=3
  Constant4 : Constant
  Data Type Conversion : DataTypeConversion
  Data Type Conversion1 : DataTypeConversion
  Data Type Conversion2 : DataTypeConversion
  Memory1 : Memory  InitialCondition=1
  Memory2 : Memory  InitialCondition=1
  Memory3 : Memory  InitialCondition=1
  MinMax : MinMax  Inputs=4
  MinMax1 : MinMax  Inputs=2
  MinMax2 : MinMax  Inputs=2
  MinMax3 : MinMax  Inputs=2
  ROOut1 : RelationalOperator  Operator===  OutDataTypeStr=boolean  RndMeth=Simplest
  ROOut2 : RelationalOperator  Operator===  OutDataTypeStr=boolean  RndMeth=Simplest
  ROOut3 : RelationalOperator  Operator===  OutDataTypeStr=boolean  RndMeth=Simplest
  Out1 : Outport
  wires:
  Data Type Conversion2/1 -> MinMax3/1
  Data Type Conversion1/1 -> MinMax2/1
  Data Type Conversion/1 -> MinMax1/1
  MinMax1/1 -> Memory1/1, MinMax/1
  MinMax2/1 -> Memory2/1, MinMax/2
  ROOut1/1 -> Data Type Conversion/1
  Memory2/1 -> MinMax2/2
  Memory3/1 -> MinMax3/2
  ROOut2/1 -> Data Type Conversion1/1
  ROOut3/1 -> Data Type Conversion2/1
  MinMax3/1 -> Memory3/1, MinMax/3
  Memory1/1 -> MinMax1/2
  [out2] -> ROOut2/2
  In1/1 -> ROOut1/1
  In2/1 -> ROOut2/1
  [out1] -> ROOut1/2
  In3/1 -> ROOut3/1
  [out3] -> ROOut3/2
  MinMax/1 -> Out1/1
  Constant4/1 -> MinMax/4

== system c00006M_harness/Eval123 ==
  In1 : Inport
  In2 : Inport  Port=2
  In3 : Inport  Port=3
  Constant4 : Constant
  Data Type Conversion : DataTypeConversion
  Data Type Conversion1 : DataTypeConversion
  Data Type Conversion2 : DataTypeConversion
  Memory1 : Memory  InitialCondition=1
  Memory2 : Memory  InitialCondition=1
  Memory3 : Memory  InitialCondition=1
  MinMax : MinMax  Inputs=4
  MinMax1 : MinMax  Inputs=2
  MinMax2 : MinMax  Inputs=2
  MinMax3 : MinMax  Inputs=2
  ROOut1 : RelationalOperator  Operator===  OutDataTypeStr=boolean  RndMeth=Simplest
  ROOut2 : RelationalOperator  Operator===  OutDataTypeStr=boolean  RndMeth=Simplest
  ROOut3 : RelationalOperator  Operator===  OutDataTypeStr=boolean  RndMeth=Simplest
  Out1 : Outport
  wires:
  Data Type Conversion2/1 -> MinMax3/1
  Data Type Conversion1/1 -> MinMax2/1
  Data Type Conversion/1 -> MinMax1/1
  MinMax1/1 -> Memory1/1, MinMax/1
  MinMax2/1 -> Memory2/1, MinMax/2
  ROOut1/1 -> Data Type Conversion/1
  Memory2/1 -> MinMax2/2
  Memory3/1 -> MinMax3/2
  ROOut2/1 -> Data Type Conversion1/1
  ROOut3/1 -> Data Type Conversion2/1
  MinMax3/1 -> Memory3/1, MinMax/3
  Memory1/1 -> MinMax1/2
  [out2] -> ROOut2/2
  In1/1 -> ROOut1/1
  In2/1 -> ROOut2/1
  [out1] -> ROOut1/2
  In3/1 -> ROOut3/1
  [out3] -> ROOut3/2
  MinMax/1 -> Out1/1
  Constant4/1 -> MinMax/4

== system c00006M_harness/Eval124 ==
  In1 : Inport
  In2 : Inport  Port=2
  In3 : Inport  Port=3
  Constant4 : Constant
  Data Type Conversion : DataTypeConversion
  Data Type Conversion1 : DataTypeConversion
  Data Type Conversion2 : DataTypeConversion
  Memory1 : Memory  InitialCondition=1
  Memory2 : Memory  InitialCondition=1
  Memory3 : Memory  InitialCondition=1
  MinMax : MinMax  Inputs=4
  MinMax1 : MinMax  Inputs=2
  MinMax2 : MinMax  Inputs=2
  MinMax3 : MinMax  Inputs=2
  ROOut1 : RelationalOperator  Operator===  OutDataTypeStr=boolean  RndMeth=Simplest
  ROOut2 : RelationalOperator  Operator===  OutDataTypeStr=boolean  RndMeth=Simplest
  ROOut3 : RelationalOperator  Operator===  OutDataTypeStr=boolean  RndMeth=Simplest
  Out1 : Outport
  wires:
  Data Type Conversion2/1 -> MinMax3/1
  Data Type Conversion1/1 -> MinMax2/1
  Data Type Conversion/1 -> MinMax1/1
  MinMax1/1 -> Memory1/1, MinMax/1
  MinMax2/1 -> Memory2/1, MinMax/2
  ROOut1/1 -> Data Type Conversion/1
  Memory2/1 -> MinMax2/2
  Memory3/1 -> MinMax3/2
  ROOut2/1 -> Data Type Conversion1/1
  ROOut3/1 -> Data Type Conversion2/1
  MinMax3/1 -> Memory3/1, MinMax/3
  Memory1/1 -> MinMax1/2
  [out2] -> ROOut2/2
  In1/1 -> ROOut1/1
  In2/1 -> ROOut2/1
  [out1] -> ROOut1/2
  In3/1 -> ROOut3/1
  [out3] -> ROOut3/2
  MinMax/1 -> Out1/1
  Constant4/1 -> MinMax/4

== system c00006M_harness/Eval126 ==
  In1 : Inport
  In2 : Inport  Port=2
  In3 : Inport  Port=3
  Constant4 : Constant
  Data Type Conversion : DataTypeConversion
  Data Type Conversion1 : DataTypeConversion
  Data Type Conversion2 : DataTypeConversion
  Memory1 : Memory  InitialCondition=1
  Memory2 : Memory  InitialCondition=1
  Memory3 : Memory  InitialCondition=1
  MinMax : MinMax  Inputs=4
  MinMax1 : MinMax  Inputs=2
  MinMax2 : MinMax  Inputs=2
  MinMax3 : MinMax  Inputs=2
  ROOut1 : RelationalOperator  Operator===  OutDataTypeStr=boolean  RndMeth=Simplest
  ROOut2 : RelationalOperator  Operator===  OutDataTypeStr=boolean  RndMeth=Simplest
  ROOut3 : RelationalOperator  Operator===  OutDataTypeStr=boolean  RndMeth=Simplest
  Out1 : Outport
  wires:
  Data Type Conversion2/1 -> MinMax3/1
  Data Type Conversion1/1 -> MinMax2/1
  Data Type Conversion/1 -> MinMax1/1
  MinMax1/1 -> Memory1/1, MinMax/1
  MinMax2/1 -> Memory2/1, MinMax/2
  ROOut1/1 -> Data Type Conversion/1
  Memory2/1 -> MinMax2/2
  Memory3/1 -> MinMax3/2
  ROOut2/1 -> Data Type Conversion1/1
  ROOut3/1 -> Data Type Conversion2/1
  MinMax3/1 -> Memory3/1, MinMax/3
  Memory1/1 -> MinMax1/2
  [out2] -> ROOut2/2
  In1/1 -> ROOut1/1
  In2/1 -> ROOut2/1
  [out1] -> ROOut1/2
  In3/1 -> ROOut3/1
  [out3] -> ROOut3/2
  MinMax/1 -> Out1/1
  Constant4/1 -> MinMax/4

== system c00006M_harness/Eval127 ==
  In1 : Inport
  In2 : Inport  Port=2
  In3 : Inport  Port=3
  Constant4 : Constant
  Data Type Conversion : DataTypeConversion
  Data Type Conversion1 : DataTypeConversion
  Data Type Conversion2 : DataTypeConversion
  Memory1 : Memory  InitialCondition=1
  Memory2 : Memory  InitialCondition=1
  Memory3 : Memory  InitialCondition=1
  MinMax : MinMax  Inputs=4
  MinMax1 : MinMax  Inputs=2
  MinMax2 : MinMax  Inputs=2
  MinMax3 : MinMax  Inputs=2
  ROOut1 : RelationalOperator  Operator===  OutDataTypeStr=boolean  RndMeth=Simplest
  ROOut2 : RelationalOperator  Operator===  OutDataTypeStr=boolean  RndMeth=Simplest
  ROOut3 : RelationalOperator  Operator===  OutDataTypeStr=boolean  RndMeth=Simplest
  Out1 : Outport
  wires:
  Data Type Conversion2/1 -> MinMax3/1
  Data Type Conversion1/1 -> MinMax2/1
  Data Type Conversion/1 -> MinMax1/1
  MinMax1/1 -> Memory1/1, MinMax/1
  MinMax2/1 -> Memory2/1, MinMax/2
  ROOut1/1 -> Data Type Conversion/1
  Memory2/1 -> MinMax2/2
  Memory3/1 -> MinMax3/2
  ROOut2/1 -> Data Type Conversion1/1
  ROOut3/1 -> Data Type Conversion2/1
  MinMax3/1 -> Memory3/1, MinMax/3
  Memory1/1 -> MinMax1/2
  [out2] -> ROOut2/2
  In1/1 -> ROOut1/1
  In2/1 -> ROOut2/1
  [out1] -> ROOut1/2
  In3/1 -> ROOut3/1
  [out3] -> ROOut3/2
  MinMax/1 -> Out1/1
  Constant4/1 -> MinMax/4

== system c00006M_harness/Eval128 ==
  In1 : Inport
  In2 : Inport  Port=2
  In3 : Inport  Port=3
  Constant4 : Constant
  Data Type Conversion : DataTypeConversion
  Data Type Conversion1 : DataTypeConversion
  Data Type Conversion2 : DataTypeConversion
  Memory1 : Memory  InitialCondition=1
  Memory2 : Memory  InitialCondition=1
  Memory3 : Memory  InitialCondition=1
  MinMax : MinMax  Inputs=4
  MinMax1 : MinMax  Inputs=2
  MinMax2 : MinMax  Inputs=2
  MinMax3 : MinMax  Inputs=2
  ROOut1 : RelationalOperator  Operator===  OutDataTypeStr=boolean  RndMeth=Simplest
  ROOut2 : RelationalOperator  Operator===  OutDataTypeStr=boolean  RndMeth=Simplest
  ROOut3 : RelationalOperator  Operator===  OutDataTypeStr=boolean  RndMeth=Simplest
  Out1 : Outport
  wires:
  Data Type Conversion2/1 -> MinMax3/1
  Data Type Conversion1/1 -> MinMax2/1
  Data Type Conversion/1 -> MinMax1/1
  MinMax1/1 -> Memory1/1, MinMax/1
  MinMax2/1 -> Memory2/1, MinMax/2
  ROOut1/1 -> Data Type Conversion/1
  Memory2/1 -> MinMax2/2
  Memory3/1 -> MinMax3/2
  ROOut2/1 -> Data Type Conversion1/1
  ROOut3/1 -> Data Type Conversion2/1
  MinMax3/1 -> Memory3/1, MinMax/3
  Memory1/1 -> MinMax1/2
  [out2] -> ROOut2/2
  In1/1 -> ROOut1/1
  In2/1 -> ROOut2/1
  [out1] -> ROOut1/2
  In3/1 -> ROOut3/1
  [out3] -> ROOut3/2
  MinMax/1 -> Out1/1
  Constant4/1 -> MinMax/4

== system c00006M_harness/Eval130 ==
  In1 : Inport
  In2 : Inport  Port=2
  In3 : Inport  Port=3
  Constant4 : Constant
  Data Type Conversion : DataTypeConversion
  Data Type Conversion1 : DataTypeConversion
  Data Type Conversion2 : DataTypeConversion
  Memory1 : Memory  InitialCondition=1
  Memory2 : Memory  InitialCondition=1
  Memory3 : Memory  InitialCondition=1
  MinMax : MinMax  Inputs=4
  MinMax1 : MinMax  Inputs=2
  MinMax2 : MinMax  Inputs=2
  MinMax3 : MinMax  Inputs=2
  ROOut1 : RelationalOperator  Operator===  OutDataTypeStr=boolean  RndMeth=Simplest
  ROOut2 : RelationalOperator  Operator===  OutDataTypeStr=boolean  RndMeth=Simplest
  ROOut3 : RelationalOperator  Operator===  OutDataTypeStr=boolean  RndMeth=Simplest
  Out1 : Outport
  wires:
  Data Type Conversion2/1 -> MinMax3/1
  Data Type Conversion1/1 -> MinMax2/1
  Data Type Conversion/1 -> MinMax1/1
  MinMax1/1 -> Memory1/1, MinMax/1
  MinMax2/1 -> Memory2/1, MinMax/2
  ROOut1/1 -> Data Type Conversion/1
  Memory2/1 -> MinMax2/2
  Memory3/1 -> MinMax3/2
  ROOut2/1 -> Data Type Conversion1/1
  ROOut3/1 -> Data Type Conversion2/1
  MinMax3/1 -> Memory3/1, MinMax/3
  Memory1/1 -> MinMax1/2
  [out2] -> ROOut2/2
  In1/1 -> ROOut1/1
  In2/1 -> ROOut2/1
  [out1] -> ROOut1/2
  In3/1 -> ROOut3/1
  [out3] -> ROOut3/2
  MinMax/1 -> Out1/1
  Constant4/1 -> MinMax/4

== system c00006M_harness/Eval131 ==
  In1 : Inport
  In2 : Inport  Port=2
  In3 : Inport  Port=3
  Constant4 : Constant
  Data Type Conversion : DataTypeConversion
  Data Type Conversion1 : DataTypeConversion
  Data Type Conversion2 : DataTypeConversion
  Memory1 : Memory  InitialCondition=1
  Memory2 : Memory  InitialCondition=1
  Memory3 : Memory  InitialCondition=1
  MinMax : MinMax  Inputs=4
  MinMax1 : MinMax  Inputs=2
  MinMax2 : MinMax  Inputs=2
  MinMax3 : MinMax  Inputs=2
  ROOut1 : RelationalOperator  Operator===  OutDataTypeStr=boolean  RndMeth=Simplest
  ROOut2 : RelationalOperator  Operator===  OutDataTypeStr=boolean  RndMeth=Simplest
  ROOut3 : RelationalOperator  Operator===  OutDataTypeStr=boolean  RndMeth=Simplest
  Out1 : Outport
  wires:
  Data Type Conversion2/1 -> MinMax3/1
  Data Type Conversion1/1 -> MinMax2/1
  Data Type Conversion/1 -> MinMax1/1
  MinMax1/1 -> Memory1/1, MinMax/1
  MinMax2/1 -> Memory2/1, MinMax/2
  ROOut1/1 -> Data Type Conversion/1
  Memory2/1 -> MinMax2/2
  Memory3/1 -> MinMax3/2
  ROOut2/1 -> Data Type Conversion1/1
  ROOut3/1 -> Data Type Conversion2/1
  MinMax3/1 -> Memory3/1, MinMax/3
  Memory1/1 -> MinMax1/2
  [out2] -> ROOut2/2
  In1/1 -> ROOut1/1
  In2/1 -> ROOut2/1
  [out1] -> ROOut1/2
  In3/1 -> ROOut3/1
  [out3] -> ROOut3/2
  MinMax/1 -> Out1/1
  Constant4/1 -> MinMax/4

== system c00006M_harness/Eval132 ==
  In1 : Inport
  In2 : Inport  Port=2
  In3 : Inport  Port=3
  Constant4 : Constant
  Data Type Conversion : DataTypeConversion
  Data Type Conversion1 : DataTypeConversion
  Data Type Conversion2 : DataTypeConversion
  Memory1 : Memory  InitialCondition=1
  Memory2 : Memory  InitialCondition=1
  Memory3 : Memory  InitialCondition=1
  MinMax : MinMax  Inputs=4
  MinMax1 : MinMax  Inputs=2
  MinMax2 : MinMax  Inputs=2
  MinMax3 : MinMax  Inputs=2
  ROOut1 : RelationalOperator  Operator===  OutDataTypeStr=boolean  RndMeth=Simplest
  ROOut2 : RelationalOperator  Operator===  OutDataTypeStr=boolean  RndMeth=Simplest
  ROOut3 : RelationalOperator  Operator===  OutDataTypeStr=boolean  RndMeth=Simplest
  Out1 : Outport
  wires:
  Data Type Conversion2/1 -> MinMax3/1
  Data Type Conversion1/1 -> MinMax2/1
  Data Type Conversion/1 -> MinMax1/1
  MinMax1/1 -> Memory1/1, MinMax/1
  MinMax2/1 -> Memory2/1, MinMax/2
  ROOut1/1 -> Data Type Conversion/1
  Memory2/1 -> MinMax2/2
  Memory3/1 -> MinMax3/2
  ROOut2/1 -> Data Type Conversion1/1
  ROOut3/1 -> Data Type Conversion2/1
  MinMax3/1 -> Memory3/1, MinMax/3
  Memory1/1 -> MinMax1/2
  [out2] -> ROOut2/2
  In1/1 -> ROOut1/1
  In2/1 -> ROOut2/1
  [out1] -> ROOut1/2
  In3/1 -> ROOut3/1
  [out3] -> ROOut3/2
  MinMax/1 -> Out1/1
  Constant4/1 -> MinMax/4

== system c00006M_harness/Eval134 ==
  In1 : Inport
  In2 : Inport  Port=2
  In3 : Inport  Port=3
  Constant4 : Constant
  Data Type Conversion : DataTypeConversion
  Data Type Conversion1 : DataTypeConversion
  Data Type Conversion2 : DataTypeConversion
  Memory1 : Memory  InitialCondition=1
  Memory2 : Memory  InitialCondition=1
  Memory3 : Memory  InitialCondition=1
  MinMax : MinMax  Inputs=4
  MinMax1 : MinMax  Inputs=2
  MinMax2 : MinMax  Inputs=2
  MinMax3 : MinMax  Inputs=2
  ROOut1 : RelationalOperator  Operator===  OutDataTypeStr=boolean  RndMeth=Simplest
  ROOut2 : RelationalOperator  Operator===  OutDataTypeStr=boolean  RndMeth=Simplest
  ROOut3 : RelationalOperator  Operator===  OutDataTypeStr=boolean  RndMeth=Simplest
  Out1 : Outport
  wires:
  Data Type Conversion2/1 -> MinMax3/1
  Data Type Conversion1/1 -> MinMax2/1
  Data Type Conversion/1 -> MinMax1/1
  MinMax1/1 -> Memory1/1, MinMax/1
  MinMax2/1 -> Memory2/1, MinMax/2
  ROOut1/1 -> Data Type Conversion/1
  Memory2/1 -> MinMax2/2
  Memory3/1 -> MinMax3/2
  ROOut2/1 -> Data Type Conversion1/1
  ROOut3/1 -> Data Type Conversion2/1
  MinMax3/1 -> Memory3/1, MinMax/3
  Memory1/1 -> MinMax1/2
  [out2] -> ROOut2/2
  In1/1 -> ROOut1/1
  In2/1 -> ROOut2/1
  [out1] -> ROOut1/2
  In3/1 -> ROOut3/1
  [out3] -> ROOut3/2
  MinMax/1 -> Out1/1
  Constant4/1 -> MinMax/4

== system c00006M_harness/Eval135 ==
  In1 : Inport
  In2 : Inport  Port=2
  In3 : Inport  Port=3
  Constant4 : Constant
  Data Type Conversion : DataTypeConversion
  Data Type Conversion1 : DataTypeConversion
  Data Type Conversion2 : DataTypeConversion
  Memory1 : Memory  InitialCondition=1
  Memory2 : Memory  InitialCondition=1
  Memory3 : Memory  InitialCondition=1
  MinMax : MinMax  Inputs=4
  MinMax1 : MinMax  Inputs=2
  MinMax2 : MinMax  Inputs=2
  MinMax3 : MinMax  Inputs=2
  ROOut1 : RelationalOperator  Operator===  OutDataTypeStr=boolean  RndMeth=Simplest
  ROOut2 : RelationalOperator  Operator===  OutDataTypeStr=boolean  RndMeth=Simplest
  ROOut3 : RelationalOperator  Operator===  OutDataTypeStr=boolean  RndMeth=Simplest
  Out1 : Outport
  wires:
  Data Type Conversion2/1 -> MinMax3/1
  Data Type Conversion1/1 -> MinMax2/1
  Data Type Conversion/1 -> MinMax1/1
  MinMax1/1 -> Memory1/1, MinMax/1
  MinMax2/1 -> Memory2/1, MinMax/2
  ROOut1/1 -> Data Type Conversion/1
  Memory2/1 -> MinMax2/2
  Memory3/1 -> MinMax3/2
  ROOut2/1 -> Data Type Conversion1/1
  ROOut3/1 -> Data Type Conversion2/1
  MinMax3/1 -> Memory3/1, MinMax/3
  Memory1/1 -> MinMax1/2
  [out2] -> ROOut2/2
  In1/1 -> ROOut1/1
  In2/1 -> ROOut2/1
  [out1] -> ROOut1/2
  In3/1 -> ROOut3/1
  [out3] -> ROOut3/2
  MinMax/1 -> Out1/1
  Constant4/1 -> MinMax/4

== system c00006M_harness/Eval136 ==
  In1 : Inport
  In2 : Inport  Port=2
  In3 : Inport  Port=3
  Constant4 : Constant
  Data Type Conversion : DataTypeConversion
  Data Type Conversion1 : DataTypeConversion
  Data Type Conversion2 : DataTypeConversion
  Memory1 : Memory  InitialCondition=1
  Memory2 : Memory  InitialCondition=1
  Memory3 : Memory  InitialCondition=1
  MinMax : MinMax  Inputs=4
  MinMax1 : MinMax  Inputs=2
  MinMax2 : MinMax  Inputs=2
  MinMax3 : MinMax  Inputs=2
  ROOut1 : RelationalOperator  Operator===  OutDataTypeStr=boolean  RndMeth=Simplest
  ROOut2 : RelationalOperator  Operator===  OutDataTypeStr=boolean  RndMeth=Simplest
  ROOut3 : RelationalOperator  Operator===  OutDataTypeStr=boolean  RndMeth=Simplest
  Out1 : Outport
  wires:
  Data Type Conversion2/1 -> MinMax3/1
  Data Type Conversion1/1 -> MinMax2/1
  Data Type Conversion/1 -> MinMax1/1
  MinMax1/1 -> Memory1/1, MinMax/1
  MinMax2/1 -> Memory2/1, MinMax/2
  ROOut1/1 -> Data Type Conversion/1
  Memory2/1 -> MinMax2/2
  Memory3/1 -> MinMax3/2
  ROOut2/1 -> Data Type Conversion1/1
  ROOut3/1 -> Data Type Conversion2/1
  MinMax3/1 -> Memory3/1, MinMax/3
  Memory1/1 -> MinMax1/2
  [out2] -> ROOut2/2
  In1/1 -> ROOut1/1
  In2/1 -> ROOut2/1
  [out1] -> ROOut1/2
  In3/1 -> ROOut3/1
  [out3] -> ROOut3/2
  MinMax/1 -> Out1/1
  Constant4/1 -> MinMax/4

== system c00006M_harness/Eval138 ==
  In1 : Inport
  In2 : Inport  Port=2
  In3 : Inport  Port=3
  Constant4 : Constant
  Data Type Conversion : DataTypeConversion
  Data Type Conversion1 : DataTypeConversion
  Data Type Conversion2 : DataTypeConversion
  Memory1 : Memory  InitialCondition=1
  Memory2 : Memory  InitialCondition=1
  Memory3 : Memory  InitialCondition=1
  MinMax : MinMax  Inputs=4
  MinMax1 : MinMax  Inputs=2
  MinMax2 : MinMax  Inputs=2
  MinMax3 : MinMax  Inputs=2
  ROOut1 : RelationalOperator  Operator===  OutDataTypeStr=boolean  RndMeth=Simplest
  ROOut2 : RelationalOperator  Operator===  OutDataTypeStr=boolean  RndMeth=Simplest
  ROOut3 : RelationalOperator  Operator===  OutDataTypeStr=boolean  RndMeth=Simplest
  Out1 : Outport
  wires:
  Data Type Conversion2/1 -> MinMax3/1
  Data Type Conversion1/1 -> MinMax2/1
  Data Type Conversion/1 -> MinMax1/1
  MinMax1/1 -> Memory1/1, MinMax/1
  MinMax2/1 -> Memory2/1, MinMax/2
  ROOut1/1 -> Data Type Conversion/1
  Memory2/1 -> MinMax2/2
  Memory3/1 -> MinMax3/2
  ROOut2/1 -> Data Type Conversion1/1
  ROOut3/1 -> Data Type Conversion2/1
  MinMax3/1 -> Memory3/1, MinMax/3
  Memory1/1 -> MinMax1/2
  [out2] -> ROOut2/2
  In1/1 -> ROOut1/1
  In2/1 -> ROOut2/1
  [out1] -> ROOut1/2
  In3/1 -> ROOut3/1
  [out3] -> ROOut3/2
  MinMax/1 -> Out1/1
  Constant4/1 -> MinMax/4

== system c00006M_harness/Eval139 ==
  In1 : Inport
  In2 : Inport  Port=2
  In3 : Inport  Port=3
  Constant4 : Constant
  Data Type Conversion : DataTypeConversion
  Data Type Conversion1 : DataTypeConversion
  Data Type Conversion2 : DataTypeConversion
  Memory1 : Memory  InitialCondition=1
  Memory2 : Memory  InitialCondition=1
  Memory3 : Memory  InitialCondition=1
  MinMax : MinMax  Inputs=4
  MinMax1 : MinMax  Inputs=2
  MinMax2 : MinMax  Inputs=2
  MinMax3 : MinMax  Inputs=2
  ROOut1 : RelationalOperator  Operator===  OutDataTypeStr=boolean  RndMeth=Simplest
  ROOut2 : RelationalOperator  Operator===  OutDataTypeStr=boolean  RndMeth=Simplest
  ROOut3 : RelationalOperator  Operator===  OutDataTypeStr=boolean  RndMeth=Simplest
  Out1 : Outport
  wires:
  Data Type Conversion2/1 -> MinMax3/1
  Data Type Conversion1/1 -> MinMax2/1
  Data Type Conversion/1 -> MinMax1/1
  MinMax1/1 -> Memory1/1, MinMax/1
  MinMax2/1 -> Memory2/1, MinMax/2
  ROOut1/1 -> Data Type Conversion/1
  Memory2/1 -> MinMax2/2
  Memory3/1 -> MinMax3/2
  ROOut2/1 -> Data Type Conversion1/1
  ROOut3/1 -> Data Type Conversion2/1
  MinMax3/1 -> Memory3/1, MinMax/3
  Memory1/1 -> MinMax1/2
  [out2] -> ROOut2/2
  In1/1 -> ROOut1/1
  In2/1 -> ROOut2/1
  [out1] -> ROOut1/2
  In3/1 -> ROOut3/1
  [out3] -> ROOut3/2
  MinMax/1 -> Out1/1
  Constant4/1 -> MinMax/4
